simulink model "TCS_Simulation"  (R2023b)
settings: Solver=FixedStepAuto  StartTime=0.0  StopTime=5  FixedStep=0.03  RelTol=1e-3
undefined symbols (not defined in the file): Ion, Lithium, sigbuilder_block
libraries: spsMosfetLib x24, fl_lib x20, nesl_utility x19, sdl_lib x12, slpidlib x5, spsBatteryLib x4, spsSeriesRLCBranchLib x4, spsPermanentMagnetSynchronousMachineLib x4, spspowerguiLib x1
(part 3 of 3)

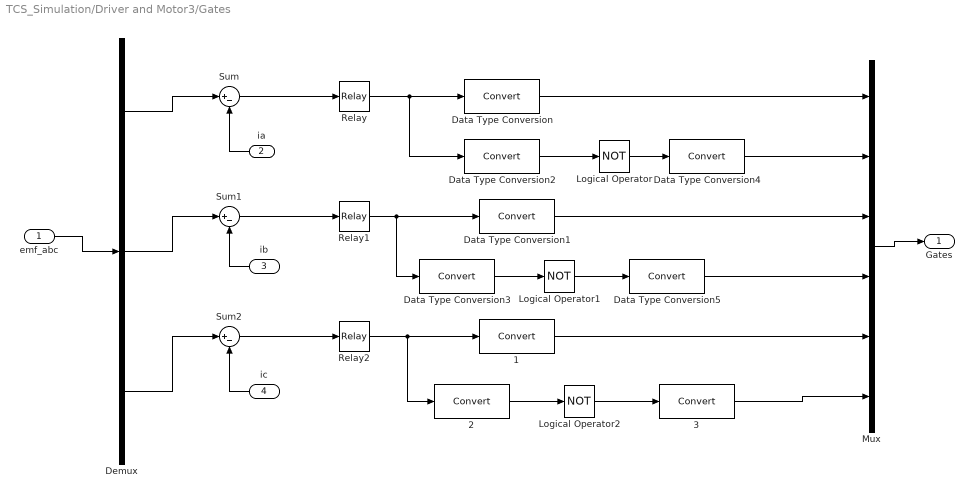
== system TCS_Simulation/Driver and Motor3/Gates ==
  emf_abc : Inport
  ia : Inport  Port=2
  ib : Inport  Port=3
  ic : Inport  Port=4
  1 : DataTypeConversion  SaturateOnIntegerOverflow=off  RndMeth=Floor
  2 : DataTypeConversion  SaturateOnIntegerOverflow=off  RndMeth=Floor
  3 : DataTypeConversion  SaturateOnIntegerOverflow=off  RndMeth=Floor
  Data Type Conversion{,1..5} (6 alike) : DataTypeConversion  SaturateOnIntegerOverflow=off  RndMeth=Floor
  Demux : Demux  Outputs=3
  Logical Operator : Logic  Operator=NOT  AllPortsSameDT=off  OutDataTypeStr=boolean
  Logical Operator1 : Logic  Operator=NOT  AllPortsSameDT=off  OutDataTypeStr=boolean
  Logical Operator2 : Logic  Operator=NOT  AllPortsSameDT=off  OutDataTypeStr=boolean
  Mux : Mux  Inputs=6
  Relay : Relay
  Relay1 : Relay
  Relay2 : Relay
  Sum : Sum  Inputs=|+-
  Sum1 : Sum  Inputs=|+-
  Sum2 : Sum  Inputs=|+-
  Gates : Outport
  wires:
  emf_abc/1 -> Demux/1
  Mux/1 -> Gates/1
  ia/1 -> Sum/2
  ib/1 -> Sum1/2
  Demux/2 -> Sum1/1
  Demux/1 -> Sum/1
  ic/1 -> Sum2/2
  Demux/3 -> Sum2/1
  Sum/1 -> Relay/1
  Sum1/1 -> Relay1/1
  Sum2/1 -> Relay2/1
  Relay/1 -> Data Type Conversion2/1, Data Type Conversion/1
  Relay1/1 -> Data Type Conversion3/1, Data Type Conversion1/1
  Relay2/1 -> 2/1, 1/1
  Data Type Conversion2/1 -> Logical Operator/1
  Data Type Conversion/1 -> Mux/1
  Data Type Conversion1/1 -> Mux/3
  Logical Operator/1 -> Data Type Conversion4/1
  Data Type Conversion4/1 -> Mux/2
  Data Type Conversion3/1 -> Logical Operator1/1
  Logical Operator1/1 -> Data Type Conversion5/1
  Data Type Conversion5/1 -> Mux/4
  1/1 -> Mux/5
  2/1 -> Logical Operator2/1
  Logical Operator2/1 -> 3/1
  3/1 -> Mux/6

== system TCS_Simulation/Driver and Motor3/Inverter ==
  Gate_signals : Inport
  Demux : Demux  Outputs=6
  Mosfet{1..6} (6 alike) : spsMosfetLib/Mosfet  Ron=0.1  Lon=0  Rd=0.01  Vfd=0  IC=0  Rs=1e5  Cs=inf  Measurements=off
  " Phase A" : PMIOPort  Side=Right
  Positive : PMIOPort  Port=2  Side=Left
  Phase B : PMIOPort  Port=3  Side=Right
  Phase C : PMIOPort  Port=4  Side=Right
  Nagative : PMIOPort  Port=5  Side=Left
  wires:
  [g1] -> Mosfet6/1
  [g2] -> Mosfet4/1
  [g3] -> Mosfet1/1
  [g4] -> Mosfet3/1
  [g5] -> Mosfet2/1
  [g6] -> Mosfet5/1
  Gate_signals/1 -> Demux/1
  Demux/1 -> [g1]
  Demux/2 -> [g2]
  Demux/3 -> [g3]
  Demux/4 -> [g4]
  Demux/5 -> [g5]
  Demux/6 -> [g6]
  connections:
  " Phase A"/RConn1 -- Mosfet4/LConn1 -- Mosfet6/RConn1
  Phase B/RConn1 -- Mosfet3/LConn1 -- Mosfet1/RConn1
  Phase C/RConn1 -- Mosfet5/LConn1 -- Mosfet2/RConn1
  Mosfet5/RConn1 -- Nagative/RConn1 -- Mosfet4/RConn1 -- Mosfet3/RConn1
  Mosfet1/LConn1 -- Mosfet6/LConn1 -- Mosfet2/LConn1 -- Positive/RConn1

== system TCS_Simulation/moment reference/High Torque ==
  Demux : Demux  Tag=STV Demux  Outputs=1
      settings: DisplayOption=none
  FromWs : FromWorkspace  Tag=STV FromWs  VariableName=tuvar
      SigBuilderData=|
      | common.afterFinalStr = 'Extrapolate'
      | common.sampleTime = 0
      | dataSet.timeRange = [0 10]
      | dataSet.name = 'Group 1'
      | sbobj.Groups.Name = 'Group 1'
      | sbobj.Groups.Signals.Name = 'Signal 1'
      | sbobj.Groups.Signals.XData = [0 0.5 1.5 2.2 4 10]
      | sbobj.Groups.Signals.YData = [0 40 120 120 120 120]
  Signal 1 : Outport  Tag=STV Outport
  wires:
  FromWs/1 -> Demux/1
  Demux/1 -> Signal 1/1

== system TCS_Simulation/moment reference1/High Torque ==
  Demux : Demux  Tag=STV Demux  Outputs=1
      settings: DisplayOption=none
  FromWs : FromWorkspace  Tag=STV FromWs  VariableName=tuvar
      SigBuilderData=|
      | common.afterFinalStr = 'Extrapolate'
      | common.sampleTime = 0
      | dataSet.timeRange = [0 10]
      | dataSet.name = 'Group 1'
      | sbobj.Groups.Name = 'Group 1'
      | sbobj.Groups.Signals.Name = 'Signal 1'
      | sbobj.Groups.Signals.XData = [0 0.5 1.5 2.2 4 10]
      | sbobj.Groups.Signals.YData = [0 40 120 120 120 120]
  Signal 1 : Outport  Tag=STV Outport
  wires:
  FromWs/1 -> Demux/1
  Demux/1 -> Signal 1/1

== system TCS_Simulation/moment reference2/High Torque ==
  Demux : Demux  Tag=STV Demux  Outputs=1
      settings: DisplayOption=none
  FromWs : FromWorkspace  Tag=STV FromWs  VariableName=tuvar
      SigBuilderData=|
      | common.afterFinalStr = 'Extrapolate'
      | common.sampleTime = 0
      | dataSet.timeRange = [0 10]
      | dataSet.name = 'Group 1'
      | sbobj.Groups.Name = 'Group 1'
      | sbobj.Groups.Signals.Name = 'Signal 1'
      | sbobj.Groups.Signals.XData = [0 0.5 1.5 2.2 4 10]
      | sbobj.Groups.Signals.YData = [0 40 120 120 120 120]
  Signal 1 : Outport  Tag=STV Outport
  wires:
  FromWs/1 -> Demux/1
  Demux/1 -> Signal 1/1
